simulink model "diagram_block_simplify1"  (R2018b)
settings: Solver=ode45  StartTime=0.0  StopTime=10.0  RelTol=1e-3  EnableMultiTasking=on
undefined symbols (not defined in the file or in its folder): f, g, Jb, Jp, ka, kb, km, l, m, Ng, r, R, s, zeta
settings Model: Creator=idan braunstain  LastModifiedBy=saar
settings DataIOCC: LimitDataPoints=on  SaveFormat=Array
settings OptimizationCC: LifeSpan=inf
settings DebuggingCC: SolverPrmCheckMsg=warning  SFUnexpectedBacktrackingDiag=warning  SFNoUnconditionalDefaultTransitionDiag=warning  SFExecutionAtInitializationDiag=none
settings HardwareCC: ProdBitPerPointer=32  ProdBitPerSizeT=32  ProdBitPerPtrDiffT=32  ProdLargestAtomicFloat=None  ProdIntDivRoundTo=Undefined  ProdEndianess=Unspecified  ProdWordSize=32  ProdHWDeviceType=32-bit Generic
settings ModelReferenceCC: PropagateSignalLabelsOutOfModel=off
settings SFSimCC: SimUseLocalCustomCode=off
settings RTWCC: RTWUseLocalCustomCode=off
settings CodeAppCC: StateflowObjectComments=on
settings GRTTargetCC: TargetLangStandard=C89/C90 (ANSI)  GeneratePreprocessorConditionals=Disable all
settings ConfigComp: CovMetricSettings=dw  CovHtmlReporting=on  CovSaveCumulativeToWorkspaceVar=on  CovSaveSingleToWorkspaceVar=on  CovExternalEMLEnable=off  CovSFcnEnable=off

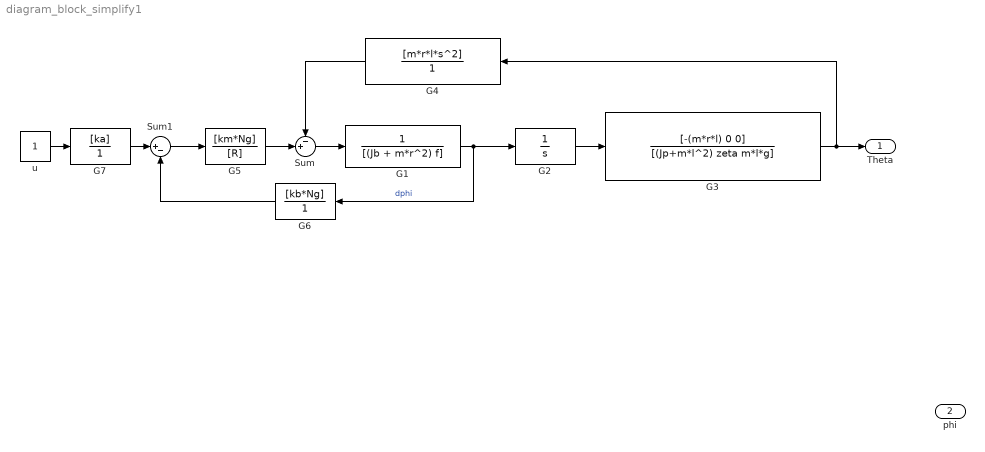
== system diagram_block_simplify1 ==
  G1 : TransferFcn  Denominator=[(Jb + m*r^2) f]
  G2 : TransferFcn  Denominator=[1 0]
  G3 : TransferFcn  Numerator=[-(m*r*l) 0 0]  Denominator=[(Jp+m*l^2) zeta m*l*g]
  G4 : TransferFcn  Numerator=[m*r*l*s^2]  Denominator=[1]
  "G5 " : TransferFcn  Numerator=[km*Ng]  Denominator=[R]
  G6 : TransferFcn  Numerator=[kb*Ng]  Denominator=[1]
  "G7 " : TransferFcn  Numerator=[ka]  Denominator=[1]
  Sum : Sum  Inputs=-+|
  Sum1 : Sum  Inputs=|+-
  u : Constant
  "Theta " : Outport
  phi : Outport  Port=2
  wires:
  "G5 "/1 -> Sum/2
  G1/1 -> G2/1, G6/1  "dphi"
  G2/1 -> G3/1
  Sum/1 -> G1/1
  G4/1 -> Sum/1
  G6/1 -> Sum1/2
  Sum1/1 -> "G5 "/1
  G3/1 -> "Theta "/1, G4/1
  u/1 -> "G7 "/1
  "G7 "/1 -> Sum1/1
